simulink model "RB_KAIROS_impControl_repulsive"  (R2020b)
settings: Solver=ode4  StartTime=0.0  StopTime=t_end  FixedStep=Ts  RelTol=1e-3
values from neighbouring files (symbols this model uses):
  am = 0.3    [RB_KAIROS_ImpControl_OpSpace_quat_2020b_safety_main.m]
  am_r = 0.3    [RB_KAIROS_ImpControl_OpSpace_quat_2020b_safety_main.m]
  Kc = diag(50*ones(6,1))    [RB_KAIROS_ImpControl_OpSpace_quat_2020b_safety_main.m]
  Kp = 2*[400;400;400;400;0;0;0]    [RB_KAIROS_ImpControl_OpSpace_quat_2020b_safety_main.m]
  Kv = [1000;1000;1000;[300;300;300;300;300;300;300]]    [RB_KAIROS_ImpControl_OpSpace_quat_2020b_safety_main.m]
  model_sample_time = 0.001    [RB_KAIROS_ImpControl_OpSpace_quat_2020b_safety_main.m]
  q_dot_0 = zeros(10,1)    [RB_KAIROS_ImpControl_OpSpace_quat_2020b_safety_main.m]
  T_i = K    [RB_KAIROS_ImpControl_OpSpace_quat_2020b_safety_main.m]
  tau_ext = [0 0 0 0 0 0 0 0 0 0 0]    [RB_KAIROS_ImpControl_OpSpace_quat_2020b_safety_main.m]
  v_SMU = 10    [RB_KAIROS_ImpControl_OpSpace_quat_2020b_safety_main.m]
  vm = 0.5    [RB_KAIROS_ImpControl_OpSpace_quat_2020b_safety_main.m]
  vm_r = 0.5    [RB_KAIROS_ImpControl_OpSpace_quat_2020b_safety_main.m]
undefined symbols (not defined in the file or in its folder): DiscIntNeverNeededParam, magnitude, q_0, T_f
libraries: simulink x4, utils x4, transformations_lib x3
(part 14 of 17)

== matlab function RB_KAIROS_impControl_repulsive/CONTROLLER /Kinematics and Dynamics/Kinematics - error representation/MATLAB Function1 ==
  data: J input; t output
function t = fcn(J)

t = 0;
%you can use normc(J) to see if one column gets near 0 and by this you get
%directions that are singular
D = sqrt(det(J*J'));
if(D < 10e-2)
    t = 1;
    disp(J)
end

== matlab function RB_KAIROS_impControl_repulsive/Trajectory Generator/Subsystem1/MATLAB Function ==
  data: u input; y output
function y = fcn(u)

y = rotm2eul(u, 'XYZ')';

== matlab function RB_KAIROS_impControl_repulsive/CONTROLLER /Kinematics and Dynamics/Kinematics - error representation/MATLAB Function2 ==
  data: R_D_W_aug input; vt output; x_dot_d input; x_ddot_d input; vt_dot output; x_err input; x_dot_err input
function [vt, vt_dot] = compute_vt(R_D_W_aug, x_dot_d, x_ddot_d, x_err, x_dot_err)
% This function is used to compute the vectors vt and vt_dot defined in Ott book in order
% to convert the equation of motion to an equivalent representation using
% error on the task variables

% INPUTS:
% - R_W_D_aug is an extension of the ROTATION MATRIX from world frame to 
%   desired frame: [R_W_D 0; 0 R_W_D], it is a 6x6 matrix
% - omega_d, p_dot_d, p_err, eps_err, omega_err are all quantities defined in
%   the world frame (or space frame) W.
S_omega_d = calc_skewsymm(x_dot_d(4:6));
S_alfa_d = calc_skewsymm(x_ddot_d(4:6));

a = [x_dot_d(1:3) + S_omega_d*(x_err(1:3));
                x_dot_d(4:6)];

vt = R_D_W_aug*a;

vt_dot = R_D_W_aug*(-augment_matrix(S_omega_d)*a + [x_ddot_d(1:3) + S_alfa_d*x_err(1:3) + S_omega_d*x_dot_err(1:3);
                                                                  x_ddot_d(4:6)]);

end 


function S = calc_skewsymm(v)

S = [0 -v(3) v(2);
    v(3) 0 -v(1);
    -v(2) v(1) 0];
end

function M_aug = augment_matrix(M)

M_aug = [M, zeros(3,3);
             zeros(3,3), M];
end

== matlab function RB_KAIROS_impControl_repulsive/CONTROLLER /Kinematics and Dynamics/Kinematics - error representation/MATLAB Function3 ==
  data: R_W_D_aug input; J_x output; J_b input
function J_x   =compute_J_x(R_W_D_aug, J_b)
% This function is used to compute the matrix J_x defined in Ott book in order
% to convert the equation of motion to an equivalent representation using
% error on the task variables

% INPUTS:
% - R_W_D_aug is an extension of the ROTATION MATRIX from world frame to 
%   desired frame: [R_W_D 0; 0 R_W_D], it is a 6x6 matrix
% - J_b is the body Jacobian of the robot 

J_x = R_W_D_aug*J_b;

== matlab function RB_KAIROS_impControl_repulsive/CONTROLLER /Kinematics and Dynamics/Kinematics - error representation/Whole-Body Jacobian ==
  data: qv input; J output size=[6,10]; qa input
function J = get_J(qv,qa)
%GET_J
%    J = GET_J(qv,qa)

%    This function was generated by the Symbolic Math Toolbox version 8.6.
%    14-Feb-2023 10:02:51

phi = qv(3);

q1 = qa(1);
q2 = qa(2);
q3 = qa(3);
q4 = qa(4);
q5 = qa(5);
q6 = qa(6);
t2 = cos(phi);
t3 = cos(q1);
t4 = cos(q2);
t5 = cos(q3);
t6 = cos(q4);
t7 = cos(q5);
t8 = cos(q6);
t9 = sin(phi);
t10 = sin(q1);
t11 = sin(q2);
t12 = sin(q3);
t13 = sin(q4);
t14 = sin(q5);
t15 = sin(q6);
t16 = t3.*t5;
t17 = t4.*t6;
t18 = t3.*t12;
t19 = t5.*t10;
t20 = t4.*t13;
t21 = t10.*t12;
t22 = -t9;
t23 = t10.*t11.*t13;
t24 = t11.*t12.*t14;
t28 = t3.*t6.*t11;
t29 = t5.*t6.*t11;
t31 = t3.*t11.*t13;
t32 = t6.*t10.*t11;
t33 = t5.*t11.*t13;
t34 = t7.*t11.*t12;
t41 = t4.*(7.9e+1./2.5e+2);
t44 = t5.*t11.*(3.3e+1./4.0e+2);
t47 = t3.*t11.*(7.9e+1./2.5e+2);
t50 = t10.*t11.*(7.9e+1./2.5e+2);
t124 = t2.*1.224646799147353e-16;
t125 = t9.*1.224646799147353e-16;
t138 = t3.*t11.*3.869883885305636e-17;
t139 = t10.*t11.*3.869883885305636e-17;
t25 = t4.*t16;
t26 = t4.*t18;
t27 = t4.*t19;
t30 = t4.*t21;
t36 = -t29;
t38 = -t31;
t39 = -t32;
t40 = -t34;
t42 = t17.*(4.8e+1./1.25e+2);
t43 = t18.*(3.3e+1./4.0e+2);
t45 = t20.*(3.3e+1./4.0e+2);
t46 = t21.*(3.3e+1./4.0e+2);
t48 = -t44;
t52 = t23.*(3.3e+1./4.0e+2);
t55 = t17+t33;
t57 = t28.*(4.8e+1./1.25e+2);
t59 = t29.*(3.3e+1./4.0e+2);
t60 = t32.*(4.8e+1./1.25e+2);
t61 = t33.*(4.8e+1./1.25e+2);
t62 = t31.*(3.3e+1./4.0e+2);
t127 = t2+t125;
t130 = t22+t124;
t132 = t28.*4.702643708725836e-17;
t133 = t32.*4.702643708725836e-17;
t136 = t18.*1.010333609296566e-17;
t137 = t21.*1.010333609296566e-17;
t141 = -t138;
t144 = t31.*1.010333609296566e-17;
t145 = t23.*1.010333609296566e-17;
t35 = -t25;
t37 = -t30;
t49 = -t45;
t51 = -t46;
t53 = t18+t27;
t54 = t19+t26;
t56 = t25.*(3.3e+1./4.0e+2);
t58 = t27.*(3.3e+1./4.0e+2);
t63 = -t52;
t65 = -t57;
t66 = -t62;
t69 = t20+t36;
t72 = t8.*t55;
t85 = t15.*t55.*(1.1e+1./1.25e+2);
t135 = -t132;
t142 = t25.*1.010333609296566e-17;
t143 = t27.*1.010333609296566e-17;
t147 = -t145;
t64 = -t56;
t67 = t16+t37;
t68 = t21+t35;
t70 = t6.*t53;
t71 = t7.*t54;
t73 = t13.*t53;
t74 = t14.*t54;
t78 = t7.*t69;
t79 = -t72;
t82 = t14.*t69;
t91 = t72.*(1.07e+2./1.0e+3);
t146 = -t142;
t75 = t6.*t68;
t76 = t7.*t67;
t77 = -t71;
t80 = t13.*t68;
t81 = t14.*t67;
t84 = t70.*(3.3e+1./4.0e+2);
t86 = t73.*(4.8e+1./1.25e+2);
t89 = t23+t70;
t94 = -t91;
t96 = t39+t73;
t97 = t24+t78;
t101 = t40+t82;
t104 = -t8.*(t32-t73);
t110 = t15.*(t32-t73).*(-1.1e+1./1.25e+2);
t112 = t15.*(t32-t73).*(1.1e+1./1.25e+2);
t114 = t8.*(t32-t73).*(-1.07e+2./1.0e+3);
t149 = t73.*4.702643708725836e-17;
t152 = t70.*1.010333609296566e-17;
t159 = t15.*(t32-t73).*(-1.077689183249671e-17);
t162 = t15.*(t32-t73).*1.077689183249671e-17;
t164 = t8.*(t32-t73).*(-1.310372075087668e-17);
t83 = -t76;
t87 = -t84;
t88 = -t86;
t90 = t75.*(3.3e+1./4.0e+2);
t92 = t80.*(4.8e+1./1.25e+2);
t98 = t28+t80;
t99 = t7.*t89;
t100 = t14.*t89;
t102 = t38+t75;
t105 = t15.*t97;
t106 = -t7.*(t31-t75);
t107 = -t14.*(t31-t75);
t109 = t8.*t97.*(1.1e+1./1.25e+2);
t150 = -t149;
t151 = t80.*4.702643708725836e-17;
t154 = -t152;
t155 = t75.*1.010333609296566e-17;
t93 = -t90;
t95 = -t92;
t103 = t8.*t98;
t108 = t15.*t98.*(1.1e+1./1.25e+2);
t115 = t105.*(1.07e+2./1.0e+3);
t117 = t81+t99;
t118 = t74+t106;
t119 = t83+t100;
t120 = t79+t105;
t122 = t77+t107;
t153 = -t151;
t156 = -t155;
t158 = t15.*t98.*1.077689183249671e-17;
t111 = -t108;
t113 = t103.*(1.07e+2./1.0e+3);
t121 = t15.*t117;
t123 = t15.*t118;
t126 = t8.*t117.*(1.1e+1./1.25e+2);
t128 = t8.*t118.*(1.1e+1./1.25e+2);
t148 = t94+t115;
t161 = -t158;
t163 = t103.*1.310372075087668e-17;
t167 = t8.*t117.*1.077689183249671e-17;
t168 = t8.*t118.*1.077689183249671e-17;
t116 = -t113;
t129 = t121.*(1.07e+2./1.0e+3);
t131 = -t128;
t134 = t123.*(1.07e+2./1.0e+3);
t157 = t104+t121;
t160 = t103+t123;
t169 = t121.*1.310372075087668e-17;
t170 = t123.*1.310372075087668e-17;
t171 = t85+t109+t148;
t140 = -t134;
t165 = t114+t129;
t166 = t113+t134;
t172 = -t157.*(t91-t115);
t174 = -t160.*(t91-t115);
t177 = t98.*t171;
t178 = -t171.*(t32-t73);
t180 = t42+t49+t59+t61+t171;
t181 = -t171.*(t76-t100);
t182 = -t171.*(t71+t14.*(t31-t75));
t183 = t171.*(t76-t100);
t199 = -t11.*t12.*(t52-t60+t84+t86+t110-t126-t129+t8.*(t32-t73).*(1.07e+2./1.0e+3));
t200 = t11.*t12.*(t52-t60+t84+t86+t110-t126-t129+t8.*(t32-t73).*(1.07e+2./1.0e+3));
t173 = -t165.*(t72-t105);
t175 = -t166.*(t72-t105);
t176 = t165.*(t72-t105);
t179 = t166.*(t72-t105);
t184 = t48+t180;
t185 = t54.*t180;
t186 = t67.*t180;
t189 = t112+t126+t165;
t191 = t111+t128+t166;
t202 = -t11.*t12.*(t57+t66+t90+t92+t108+t116+t131+t140);
t203 = t11.*t12.*(t57+t66+t90+t92+t108+t116+t131+t140);
t210 = -t4.*(t51+t56+t57+t66+t90+t92+t108+t116+t131+t140);
t211 = t47+t51+t56+t57+t66+t90+t92+t108+t116+t131+t140;
t187 = t3.*t11.*t184;
t188 = t10.*t11.*t184;
t192 = t41+t184;
t193 = t55.*t189;
t194 = t55.*t191;
t195 = -t189.*(t34-t82);
t196 = -t191.*(t34-t82);
t197 = t191.*(t34-t82);
t198 = t60+t63+t87+t88+t189;
t201 = t62+t65+t93+t95+t191;
t206 = t172+t176;
t208 = t174+t179;
t216 = t186+t200;
t217 = t185+t203;
t220 = t133+t136+t139+t143+t147+t150+t154+t162+t164+t167+t169+t211+1.1e+1./4.0e+1;
t190 = -t188;
t204 = t43+t58+t198;
t207 = t46+t64+t201;
t212 = t178+t193;
t213 = t177+t194;
t214 = t183+t195;
t215 = t182+t197;
t219 = t187+t210;
t205 = t4.*t204;
t209 = t50+t204;
t218 = t190+t205;
t221 = t135+t137+t141+t144+t146+t153+t156+t161+t163+t168+t170+t209+3.1e+1./2.0e+2;
J = reshape([1.0,0.0,0.0,0.0,0.0,0.0,0.0,1.0,0.0,0.0,0.0,0.0,t2.*t221+t9.*t220,-t2.*t220+t9.*t221,0.0,0.0,0.0,1.0,t127.*t209-t130.*t211,-t127.*t211-t130.*t209,0.0,0.0,0.0,1.0,-t3.*t127.*t192-t10.*t130.*t192,t3.*t130.*t192-t10.*t127.*t192,-t3.*t211-t10.*t209,-t3.*t130+t10.*t127,-t3.*t127-t10.*t130,0.0,t130.*t219-t127.*(t188-t205),t127.*t219+t130.*(t188-t205),-t10.*t11.*(t51+t56+t57+t66+t90+t92+t108+t116+t131+t140)+t3.*t11.*t204,-t3.*t11.*t127-t10.*t11.*t130,t3.*t11.*t130-t10.*t11.*t127,t4,t127.*t216+t130.*t217,t127.*t217-t130.*t216,t67.*(t57+t66+t90+t92+t108+t116+t131+t140)-t54.*(t52-t60+t84+t86+t110-t126-t129+t8.*(t32-t73).*(1.07e+2./1.0e+3)),-t54.*t127+t67.*t130,t54.*t130+t67.*t127,-t11.*t12,t127.*(t193-t171.*(t32-t73))+t130.*t213,-t130.*(t193-t171.*(t32-t73))+t127.*t213,t98.*t189+t191.*(t32-t73),-t98.*t127-t130.*(t32-t73),t98.*t130-t127.*(t32-t73),t55,t127.*t214+t130.*(t196+t171.*(t71+t14.*(t31-t75))),-t130.*t214+t127.*(t196+t171.*(t71+t14.*(t31-t75))),t189.*(t71+t14.*(t31-t75))-t191.*(t76-t100),-t127.*(t71+t14.*(t31-t75))+t130.*(t76-t100),t130.*(t71+t14.*(t31-t75))+t127.*(t76-t100),t101,-t127.*t206-t130.*t208,-t127.*t208+t130.*t206,t157.*t166-t160.*t165,t127.*t160-t130.*t157,-t127.*t157-t130.*t160,t120],[6,10]);

== matlab function RB_KAIROS_impControl_repulsive/CONTROLLER /MATLAB Function ==
  data: qa_des input; qa_des_new output; qv input
function qa_des_new = fcn(qa_des,qv)

qa_des_new = qa_des;
% qa_des_new(1) = qa_des_new(1)+qv(3);

== matlab function RB_KAIROS_impControl_repulsive/CONTROLLER /Primary task - Controller/MATLAB Function ==
  data: Kc input; Dc output; Lambda input
function Dc = compute_damping(Kc,Lambda)
%  COMPUTE_DAMPING Computes damping matrix to enforce desired second order
%  system behaviour.
%
%   Dc = COMPUTE_DAMPING(Kc,Lambda) computes the damping depending on 
%        stiffness matrix Kc (which has to be constant for stability) and
%        inertia matrix Lambda (which is time varying since no inertia 
%        shaping is applied).
%   
%   Reference: Cartesian Impedance Control of Redundant and Flexible-Joint
%              Robots, C. Ott 2005, page 36-37.
%   See also EIG

% % DAMPING MATRIX (varying) simplified
zeta = 1*ones(6,1);

A = real(sqrtm(Lambda));
Kc_1 = real(sqrtm(Kc));
D0 = diag(zeta);
Dc = A*D0*Kc_1 + Kc_1*D0*A;

% DAMPING MATRIX (varying)
%Generalized eigenvalue decomposition for the pair (Kc,Lambda)
% [eigvecs,eigvals] = eig(Kc, Lambda);
% eigvals = real(eigvals);
% eigvecs = real(eigvecs);
% %sorting eigs by magnitude
% %[eigvals,sidx] = sort(diag(eigvals),'descend');
% 
% %Finding matrices that satisfy K = Q'K0Q and Lambda = Q'*Q
% K0 = eigvals;
% %V = eigvecs(:,sidx);
% Q_T = Lambda*eigvecs;
% Q = Q_T';
% 
% %Damping matrix computation
% zeta = 1*ones(6,1); %Imposing an overdamped behaviour
% D0 = diag(zeta).*K0;
% Dc = 2*Q_T*D0*Q;

%OLD implementation where stiffness and damping were retrieven from
%configuration parameters
%function [Kc,Dc] = compute_stiffness_damping(J, J_T, J_i, J_d, Lambda)

% Kq_veh = [750*ones(2,1); 750]; 
% Dq_veh = [800;800;800];
% Kq_arm = [350;250;100;170;50;20;10];
% Dq_arm = [60;200;120;150;20;30;5];
% 
% Kq = diag([Kq_veh;Kq_arm]);
% Dq = diag([Dq_veh;Dq_arm]);
% 
% Dc = J_i'*Dq*J_i;
% Kc = J_i'*(Kq-J_T*Dc*J_d)*J_i;

% Kc = diag([150;180;105;1.5;15;52.5]);
% Dc = diag([180;200;80;10;10;6]);

== matlab function RB_KAIROS_impControl_repulsive/CONTROLLER /Secondary task - Controller/MATLAB Function ==
  data: qa_des input; qa input; tau_n output; qa_dot input; qv_dot input; M input; J_x_T input; J_x_i input; Kp input; Kv input
function tau_n = compute_null_space_torque(qa_des, qa, qa_dot, qv_dot, M, J_x_T, J_x_i, Kp, Kv)


%% Version 1: Try to keep the robot joints in their mid position
% q_max = [2.3093; 1.5133; 2.4937; -0.4461; 2.4800; 4.2094; 2.6895];
% q_min = [-2.3093; -1.5133; -2.4937; -2.7478; -2.4800; 0.8521; -2.6895];
% tau_0 = -M*[Kv(1:3).*qv_dot;2*Kp.*(qa-(q_max+q_min)./2)+Kv(4:10).*qa_dot];
% Good but the mid config. of every joint is not super good for any motion

%% Version 2: Mantain a certain configuration 
%Compute generalized joint torque based on the gradient of the potential
%that is used to mantain a certain configuration of the arm.

    tau_0 = -M*[Kv(1:3).*qv_dot;
         Kp.*(qa-qa_des)+Kv(4:10).*qa_dot]; 
    

%% Projection of the torque in the null space
tau_n = (eye(size(M,2))-J_x_T*J_x_i')*tau_0;

== matlab function RB_KAIROS_impControl_repulsive/EE to task space quaternion quantities/Augment matrix ==
  data: R_W_D input; R_D_W_aug output
function R_D_W_aug = augment_matrix(R_W_D)

R_D_W_aug = [R_W_D', zeros(3,3);
             zeros(3,3), R_W_D'];

== matlab function RB_KAIROS_impControl_repulsive/EE to task space quaternion quantities/Get Pose in quaternions ==
  data: T_W_EE input; p_EE output; qt_EE output
function [p_EE, qt_EE] = tform2pose_quat(T_W_EE)
% Retrieves the pose of the end effector using quaternion representation
% for the orientation 

p_EE = T_W_EE(1:3,4);
qt_EE = tform2quat(T_W_EE)';

== matlab function RB_KAIROS_impControl_repulsive/Trajectory Generator/move2pose/Cartesian_ipol2/rotation/Embedded MATLAB Function1 ==
  data: t input; qd output; s0 input; v0 input; sf input; vm input; am input; dqd output; ddqd output; ipol_finished output; T_scale input; interpoly input
function [qd,dqd,ddqd, ipol_finished] = calc_qd(t,s0,v0,sf,vm,am,T_scale,interpoly)
% This function calculates a one dimensional movement with a trapezodial 
% signal for velocity over time. Additionally it is able to adapt to shifts
% in the maximum allowed velocity.
%
% Inputs:
% t         current runtime
% s0        start value for motion in position
% v0        start value for motion in velocity
% sf        final value for motion in position
% vm        maximum allowed velocity
% am        maximum allowed acceleration
% T_scale   Scaling factor for duration of adaption
% interpoly Which interpolation to use
%
% Outputs:
% qd        disered position at current time
% dqd       disered velocity at current time
% ddqd      disered acceleration at current time
% ipol_finished 
%           motion is finished

%% Initialize persistent variables for adaption motion
persistent vm1 adpt ti qi qf T t_shift
if isempty(vm1)
    vm1 = vm;       %remembers the max velocity from last run
end
if isempty(adpt)
    adpt = false;   %stores if an adaption motion is activated
end
if isempty(ti)
    ti = 0;         %Initial time step for adaption motion
end
if isempty(qi)
    qi = zeros(3,1);%Initial values (pos,vel,acc) for adaption motion
end
if isempty(qf)
    qf = zeros(3,1);%Final values (pos,vel,acc) for adaption motion
end
if isempty(T)
    T = 0;          %Duration of adaption motion; tf = ti+T
end
if isempty(t_shift)
    t_shift = 0;    %Time distance with which the current reference motion is shifted
end

% needed to delay tanhlog with one timestep
tanhlog_delay = 0;

%% This If runs only for one timestep!!!
% If current max velocity is unequal to old one 
% Not directly at the beginning
% Dont start new while a adaption is still running, to prevent reset of
%   initial values
if abs(vm-vm1)>1e-3 && t>0.001 && adpt==false                       
    adpt = true;          % Activate adaption
    ti = t;               % Set initial timestep to current step
    tanhlog_delay = 1;    % Activate the delay for tanhlog

    %%% inital set of position, velo, acceleration for adaption motion 
    % is the same as the old mogen would do (t_shift is not updated at
    % this time!)
    [qi, ~] = interpolator(ti+t_shift, compute_traj_parameters(s0, v0, sf, vm1, am));

    %%% computes the time shift for shifting the new motion to the end
    % point of the old motion. So at which time the new motion has
    % the same qd? Then calculate the time distance to the inital
    % time of the change in velocities
    % t_shift < 0 if new motion is faster (vm>vm1)
    % t_shift > 0 if new motion is slower (vm<vm1)
    % interpolator_1 is the inverse function of interpolator!
    t_shift = interpolator_1(qi(1), compute_traj_parameters(s0, v0, sf, vm, am)) - ti ;

    %%% Additional shift for adaption motion = Duration of adaption motion
    T_standard = abs(vm1-vm)/am;
    switch interpoly
        case 0
            T = 0;
            adpt = false;       %no adatption  
        case 1
            T = T_standard*2.2;    %tanhlog
        case 2
            T = (pi*abs(vm1-vm))/(2*am);  %Cosine version
        case 3
            T = T_standard;        %poly3
        case 4
            T = 1.5*(abs(vm1-vm)/am); %poly4
        case 5
            T = T_standard*1.5;        %poly5 
        case 7
            T = T_standard*1.75;        %poly7 
        otherwise
            T = T_standard;        %rest
    end

    % Scale Duration if needed
    T = T*T_scale;

    %%% The additional shift for adaption motion is dependent on the
    % difference in the velocities. See report for details.
    t_shift  = t_shift+(T/2)*((vm1/vm)-1);

    %%% Calculate final values for adaption motion. Which are reached
    % at inital time plus duration of adaption and new time shift
    [qf, ~] = interpolator(ti+t_shift+T, compute_traj_parameters(s0, v0, sf, vm, am));

end

%% Here the actual motion is calculated
% Interpolates the values of pos,vel,acc (qv) with parameters and current time t    
[qdv, ipol_finished] = interpolator(t+t_shift, compute_traj_parameters(s0, v0, sf, vm, am));  

%% If adaption motion needed
if adpt == true 

    %%% calculate the adaption moition, which takes time from ti to
    % ti+T. t is the current runtime, _i initial values, _f final
    % values, _m maximum values

    switch interpoly
        case 0
            adpt=false;                             %no adatption  
        case 1
            if tanhlog_delay == 1
                qdv = qi;  
                tanhlog_delay = 0;
            else
                qdv = tanhlog(t,ti,T,qi,qf,vm,am);      %tanhlog
            end
        case 2
            qdv = cosine(t,ti,T,qi,qf,vm,am);       %Cosine version
        case 3
            qdv = poly3(t,ti,T,qi,qf,vm,am);        %poly3
        case 4
            qdv = poly4(t,ti,T,qi,qf,vm,am);        %poly4
        case 5
            qdv = poly5(t,ti,T,qi,qf,vm,am);        %poly5 
        case 6
            qdv = poly6(t,ti,T,qi,qf,vm,am);        %poly6 
        case 7
            qdv = poly7(t,ti,T,qi,qf,vm,am);        %poly7 
        case 8
            qdv = poly4_mean(t,ti,T,qi,qf,vm,am);   %poly4_mean 
        case 9
            qdv = poly5_2mean(t,ti,T,qi,qf,vm,am);  %poly5_2mean 
        case 10
            qdv = tanhmean(t,ti,T,qi,qf,vm,am);     %tanhmean 
        otherwise
            error('Unknown adaption motion');       %rest
    end

    % If time is equal than the finish time => adaption motion is complete
    % But it is aborted one timestep earlier, since the finish timestep
    % is already computed correctly by the standard interpolator.
    if t >= (ti+T-0.001)
        adpt = false;     % If adaption finished => reset
    end
end

%% Set output
if sf == s0          % No motion needed if start = end 
    qd = s0;         % => set initial values
    dqd = v0;
    ddqd = 0;  
else     
    qd = qdv(1);     % set output
    dqd = qdv(2);
    ddqd = qdv(3);        
end

vm1 = vm;  %remember current max velocity

end

function [qv] = poly3(t,ti,T,qvi,qvf,dqm,ddqm)
%POLY3 computes a polynomial trajectory of degree 3 between initial (_i) 
%values and final (_f) values of position q, velocity dq and accelerataion
%ddq. Taken from Melchiorri presentation page 19

qi = qvi(1);      %split input vectors in pos,vel,acc
dqi = qvi(2);
ddqi = qvi(3);
qf = qvf(1);
dqf = qvf(2);
ddqf = qvf(3);
      
% current duration of motion dt
dt = t-ti;                      

% compute coefficients
a0 = qi;
a1 = dqi;
a2 = (-3*(qi-qf)-(2*dqi+dqf)*T)/(T^2);
a3 = (2*(qi-qf)+(dqi+dqf)*T)/(T^3);

% compute pos,vel,acc desired (_d)
qd = a0+a1*dt+a2*dt^2+a3*dt^3;
dqd = a1+2*a2*dt+3*a3*dt^2;
ddqd = 2*a2+6*a3*dt;

qv = [qd;dqd;ddqd]; %Send values back

end

function [qv] = poly4(t,ti,T,qvi,qvf,dqm,ddqm)
%POLY4 computes a polynomial trajectory of degree 4 between initial (_i) 
%values and final (_f) values of position q, velocity dq and accelerataion
%ddq. inspired by old function in here

qi = qvi(1);      %split input vectors in pos,vel,acc
dqi = qvi(2);
ddqi = qvi(3);
qf = qvf(1);
dqf = qvf(2);
ddqf = qvf(3);
      
% current duration of motion dt
dt = t-ti;                      

% a2 = 0;
% a3 = -4/9*ddqm^2/(dqi-dqm);
% a4 = -4/27*ddqm^3/(dqi-dqm)^2;
a2 = 0;
a3 = -4/9*ddqm^2/abs(dqi-dqf);
a4 = 4/27*ddqm^3/abs(dqi-dqf)^2;

a0 = qi;
a1 = dqi;
% a2 = 0.5*ddqi;
% a3 = (4*(qf-qi)-(dqf+3*dqi)*T-ddqi*(T^2))/(T^3);
% a4 = (3*(qi-qf)+(dqf+2*dqi)*T+0.5*ddqi*(T^2))/(T^4);

% compute pos,vel,acc desired (_d)
qd = (a4*dt^4+a3*dt^3+a2*dt^2+a1*dt+a0);
dqd = 4*a4*dt^3+3*a3*dt^2+2*a2*dt+a1;
ddqd = 12*a4*dt^2+6*a3*dt+2*a2;

qv = [qd;dqd;ddqd]; %Send values back

end

function [qv] = poly4_mean(t,ti,T,qvi,qvf,dqm,ddqm)
%POLY4 computes a polynomial trajectory of degree 4 between initial (_i) 
%values and final (_f) values of position q, velocity dq and accelerataion
%ddq with mean velocity at T/2. self made

qi = qvi(1);      %split input vectors in pos,vel,acc
dqi = qvi(2);
ddqi = qvi(3);
qf = qvf(1);
dqf = qvf(2);
ddqf = qvf(3);
      
% current duration of motion dt
dt = t-ti;                     

b = [qi dqi qf dqf 0.5*(dqi+dqf)]';

M_inv = [...
       1,     0,      0,          0,           0;
       0,     1,      0,          0,           0;
   6/T^2,  -2/T, -6/T^2,    5/(4*T),    27/(4*T);
 -16/T^3, 1/T^2, 16/T^3, -7/(2*T^2), -27/(2*T^2);
   9/T^4,     0, -9/T^4,  9/(4*T^3),  27/(4*T^3)];

a = M_inv * b;

% compute pos,vel,acc desired (_d)

qd = a(1)+a(2)*dt+a(3)*dt^2+a(4)*dt^3+a(5)*dt^4;
dqd = a(2)+2*a(3)*dt+3*a(4)*dt^2+4*a(5)*dt^3;
ddqd = 2*a(3)+6*a(4)*dt+12*a(5)*dt^2;

qv = [qd;dqd;ddqd]; %Send values back

end

function [qv] = poly5(t,ti,T,qvi,qvf,dqm,ddqm)
%POLY5 computes a polynomial trajectory of degree 5 between initial (_i) 
%values and final (_f) values of position q, velocity dq and accelerataion
%ddq. Taken from Melchiorri presentation page 25

qi = qvi(1);      %split input vectors in pos,vel,acc
dqi = qvi(2);
ddqi = qvi(3);
qf = qvf(1);
dqf = qvf(2);
ddqf = qvf(3);
      
% current duration of motion dt
dt = t-ti;                      

% compute coefficients
a0 = qi;
a1 = dqi;
a2 = 0.5*ddqi;
a3 = (20*(qf-qi)-(8*dqf+12*dqi)*T-(3*ddqf-ddqi)*T^2)/(2*T^3);
a4 = (30*(qi-qf)+(14*dqf+16*dqi)*T+(3*ddqf-2*ddqi)*T^2)/(2*T^4);
a5 = (12*(qf-qi)-6*(dqf+dqi)*T-(ddqf-ddqi)*T^2)/(2*T^5);

% compute pos,vel,acc desired (_d)
qd = a0+a1*dt+a2*dt^2+a3*dt^3+a4*dt^4+a5*dt^5;
dqd = a1+2*a2*dt+3*a3*dt^2+4*a4*dt^3+5*a5*dt^4;
ddqd = 2*a2+6*a3*dt+12*a4*dt^2+20*a5*dt^3;

qv = [qd;dqd;ddqd]; %Send values back

end

function [qv] = poly5_2mean(t,ti,T,qvi,qvf,dqm,ddqm)
%POLY5 computes a polynomial trajectory of degree 5 between initial (_i) 
%values and final (_f) values of position q, velocity dq and accelerataion
%ddq with 2*mean steps at T/3 and 2T/3. self made

qi = qvi(1);      %split input vectors in pos,vel,acc
dqi = qvi(2);
ddqi = qvi(3);
qf = qvf(1);
dqf = qvf(2);
ddqf = qvf(3);
      
% current duration of motion dt
dt = t-ti;                      

% compute coefficients
b = [qi dqi qf dqf 0.5*(dqi+dqf)+(1/6)*(dqi-dqf) 0.5*(dqi+dqf)+(1/6)*(dqi-dqf)]';

M_inv = [...
        1,          0,        0,           0,            0,           0;
        0,          1,        0,           0,            0,           0;
  -30/T^2,  -13/(2*T),   30/T^2,   -13/(4*T),    -27/(4*T),   -27/(2*T);
  110/T^3, 67/(4*T^2), -110/T^3,  49/(4*T^2),  135/(4*T^2), 189/(4*T^2);
 -135/T^4,    -18/T^3,  135/T^4, -63/(4*T^3), -189/(4*T^3),     -54/T^3;
   54/T^5, 27/(4*T^4),  -54/T^5,  27/(4*T^4),   81/(4*T^4),  81/(4*T^4)];

a = M_inv * b;

% compute pos,vel,acc desired (_d)

qd = a(1)+a(2)*dt+a(3)*dt^2+a(4)*dt^3+a(5)*dt^4+a(6)*dt^5;
dqd = a(2)+2*a(3)*dt+3*a(4)*dt^2+4*a(5)*dt^3+5*a(6)*dt^4;
ddqd = 2*a(3)+6*a(4)*dt+12*a(5)*dt^2+20*a(6)*dt^3;

qv = [qd;dqd;ddqd]; %Send values back

end

function [qv] = poly6(t,ti,T,qvi,qvf,dqm,ddqm)
%POLY6 computes a polynomial trajectory of degree 6 between initial (_i) 
%values and final (_f) values of position q, velocity dq and accelerataion
%ddq with mean velocity at T/3. self made

qi = qvi(1);      %split input vectors in pos,vel,acc
dqi = qvi(2);
ddqi = qvi(3);
qf = qvf(1);
dqf = qvf(2);
ddqf = qvf(3);

% current duration of motion dt
dt = t-ti;                      

% compute coefficients
b = [qi dqi 0.5*ddqi qf dqf ddqf 0.5*(dqi+dqf)]';

M_inv = [...
       1,      0,      0,       0,           0,          0,            0;
       0,      1,      0,       0,           0,          0,            0;
       0,      0,      1,       0,           0,          0,            0;
  20/T^3, -6/T^2,   -4/T, -20/T^3,  23/(4*T^2),   -1/(2*T),   81/(4*T^2);
 -75/T^4,  8/T^3,  6/T^2,  75/T^4, -89/(4*T^3),      2/T^2, -243/(4*T^3);
  84/T^5, -3/T^4, -4/T^3, -84/T^5, 105/(4*T^4), -5/(2*T^3),  243/(4*T^4);
 -30/T^6,      0,  1/T^4,  30/T^6, -39/(4*T^5),      1/T^4,  -81/(4*T^5)];

a = M_inv * b;

% compute pos,vel,acc desired (_d)

qd = a(1)+a(2)*dt+a(3)*dt^2+a(4)*dt^3+a(5)*dt^4+a(6)*dt^5+a(7)*dt^6;
dqd = a(2)+2*a(3)*dt+3*a(4)*dt^2+4*a(5)*dt^3+5*a(6)*dt^4+6*a(7)*dt^5;
ddqd = 2*a(3)+6*a(4)*dt+12*a(5)*dt^2+20*a(6)*dt^3+30*a(7)*dt^4;

qv = [qd;dqd;ddqd]; %Send values back

end

function [qv] = poly7(t,ti,T,qvi,qvf,dqm,ddqm)
%POLY7 computes a polynomial trajectory of degree 7 between initial (_i) 
%values and final (_f) values of position q, velocity dq, accelerataion
%ddq and jerk dddq. self made

qi = qvi(1);      %split input vectors in pos,vel,acc
dqi = qvi(2);
ddqi = qvi(3);
dddqi = 0;
qf = qvf(1);
dqf = qvf(2);
ddqf = qvf(3);
dddqf = 0;

% current duration of motion dt
dt = t-ti;                      

% compute coefficients
 
a = [...
                                                                                                                                                                            conj(qi)
                                                                                                                                                                           conj(dqi)
                                                                                                                                                                        conj(ddqi)/2
                                                                                                                                                                       conj(dddqi)/6
           (5*conj(ddqf))/(2*T^2) - (2*conj(dddqi))/(3*T) - conj(dddqf)/(6*T) - (5*conj(ddqi))/T^2 - (15*conj(dqf))/T^3 - (20*conj(dqi))/T^3 + (35*conj(qf))/T^4 - (35*conj(qi))/T^4
                  conj(dddqf)/(2*T^2) + conj(dddqi)/T^2 - (7*conj(ddqf))/T^3 + (10*conj(ddqi))/T^3 + (39*conj(dqf))/T^4 + (45*conj(dqi))/T^4 - (84*conj(qf))/T^5 + (84*conj(qi))/T^5
 (13*conj(ddqf))/(2*T^4) - (2*conj(dddqi))/(3*T^3) - conj(dddqf)/(2*T^3) - (15*conj(ddqi))/(2*T^4) - (34*conj(dqf))/T^5 - (36*conj(dqi))/T^5 + (70*conj(qf))/T^6 - (70*conj(qi))/T^6
               conj(dddqf)/(6*T^4) + conj(dddqi)/(6*T^4) - (2*conj(ddqf))/T^5 + (2*conj(ddqi))/T^5 + (10*conj(dqf))/T^6 + (10*conj(dqi))/T^6 - (20*conj(qf))/T^7 + (20*conj(qi))/T^7];
 


% compute pos,vel,acc desired (_d)

qd = a(1)+a(2)*dt+a(3)*dt^2+a(4)*dt^3+a(5)*dt^4+a(6)*dt^5+a(7)*dt^6+a(8)*dt^7;
dqd = a(2)+2*a(3)*dt+3*a(4)*dt^2+4*a(5)*dt^3+5*a(6)*dt^4+6*a(7)*dt^5+7*a(8)*dt^6;
ddqd = 2*a(3)+6*a(4)*dt+12*a(5)*dt^2+20*a(6)*dt^3+30*a(7)*dt^4+42*a(8)*dt^5;

qv = [qd;dqd;ddqd]; %Send values back

end

function [qv] = cosine(t,ti,T,qvi,qvf,dqm,ddqm)
%COSINE computes a cosine trajectory between initial (_i) 
%values and final (_f) values of position q, velocity dq and accelerataion
%ddq with respect to the maximum values (_m). t is the current runtime

qi = qvi(1);      %split input vectors in pos,vel,acc
dqi = qvi(2);
ddqi = qvi(3);
qf = qvf(1);
dqf = qvf(2);
ddqf = qvf(3);
      
% often needed values

%T = (pi*abs(dqf-dqi))/(2*ddqm); % total duration of motion T (with am)
%T = abs((2*(qf-qi))/(dqi-dqf));
dt = t-ti;                      % current duration of motion dt

%cm = (T/(2*pi))*(dqm-(1/T)*(qf-qi));
c = qi-0.5*(dqi+dqf)*ti;
%cn = qf-0.5*(dqi+dqf)*(ti+T);
%c = cn + 0.5*(1+cos((pi/T)*dt))*(ca-cn);


% if t<(ti+(T/2))
%     c = qi - 0.5*(dqi+dqf)*ti;
% else
%     c = qf - 0.5*(((dqi+dqf)/2)+dqf)*tf;
% end

%c = (qi+qf)/2 - 0.5*(dqi+dqf)*(ti+(T/2)) - 0.5*(dqi-dqf)*(T/pi);
% compute pos,vel,acc desired (_d)
%qd = qi + (1/T)*(qf-qi)*dt + cm*sin(((2*pi)/T)*dt);
qd = 0.5*(dqi+dqf)*t + 0.5*(T/pi)*(dqi-dqf)*sin((pi/T)*dt) + c;
dqd = 0.5*(dqi+dqf) + 0.5*(dqi-dqf)*cos((pi/T)*dt);
ddqd = -0.5*(pi/T)*(dqi-dqf)*sin((pi/T)*dt);

qv = [qd;dqd;ddqd]; %Send values back

end

function [qv] = tanhmean(t,ti,T,qvi,qvf,dqm,ddqm)
%TANHMEAN computes a tanh trajectory between initial (_i) 
%values and final (_f) values of position q, velocity dq and accelerataion
%ddq with respect to the maximum values (_m). t is the current runtime
%selfmade

qi = qvi(1);      %split input vectors in pos,vel,acc
dqi = qvi(2);
ddqi = qvi(3);
qf = qvf(1);
dqf = qvf(2);
ddqf = qvf(3);
      
% current duration of motion dt
dt = t-ti;                      
t_norm = dt/T;
theta = 4;

qd = 0.5*(1/theta)*(dqf-dqi)*log(cosh(theta*(t_norm-0.5))) ...
     + 0.5*(dqi+dqf)*t_norm ...
     + qf - 0.5*(1/theta)*(dqf-dqi)*log(cosh(0.5*theta));
     %+ qi - 0.5*(1/theta)*(dqf-dqi)*log(cosh(-0.5*theta));
dqd = 0.5*(dqi+dqf) + 0.5*(dqf-dqi)*tanh(theta*(t_norm-0.5));
ddqd = 0.5*theta*(dqf-dqi)*sech(t_norm-0.5)^2;

qv = [qd;dqd;ddqd]; %Send values back

end

function [qv] = tanhlog(t,ti,T,qvi,qvf,dqm,ddqm)
%TANHLOG computes a tanh-log trajectory between initial (_i) 
%values and final (_f) values of position q, velocity dq and accelerataion
%ddq with respect to the maximum values (_m). t is the current runtime
%taken from Internet

qi = qvi(1);      %split input vectors in pos,vel,acc
dqi = qvi(2);
ddqi = qvi(3);
qf = qvf(1);
dqf = qvf(2);
ddqf = qvf(3);
      
% current duration of motion dt
dt = t-ti;  

a = dqi;
b = qi;      
c = dqf;
d = qf-dqf*T;
k = d-b;

x = (a*dt+b-c*dt-d+k)/(2*k);
w = (tanh(((log(1-x))^2-(log(x))^2)/3)+1)/2;
p = tanh((log(2-x)-log(x))*(1-(1/sqrt(2))*(log(2-x)+log(x))))+2*x-1;
q = tanh((log(x+1)-log(1-x))*(1-(1/sqrt(2))*(log(1-x)+log(x+1))));
s = p*(1-w)+q*w;

qd = k*s+c*dt+d-k;

dqd = dqf + (qi - qf + T*dqf)*((tanh(log((dqf*dt - dqi*dt)/(2*qi - 2*qf + 2*T*dqf))^2/3 - log(1 - (dqf*dt - dqi*dt)/(2*qi - 2*qf + 2*T*dqf))^2/3)/2 + 1/2)*((((2^(1/2)*(log(2 - (dqf*dt - dqi*dt)/(2*qi - 2*qf + 2*T*dqf)) + log((dqf*dt - dqi*dt)/(2*qi - 2*qf + 2*T*dqf))))/2 - 1)*((dqf - dqi)/(dqf*dt - dqi*dt) - (dqf - dqi)/(((dqf*dt - dqi*dt)/(2*qi - 2*qf + 2*T*dqf) - 2)*(2*qi - 2*qf + 2*T*dqf))) - (2^(1/2)*(log(2 - (dqf*dt - dqi*dt)/(2*qi - 2*qf + 2*T*dqf)) - log((dqf*dt - dqi*dt)/(2*qi - 2*qf + 2*T*dqf)))*((dqf - dqi)/(dqf*dt - dqi*dt) + (dqf - dqi)/(((dqf*dt - dqi*dt)/(2*qi - 2*qf + 2*T*dqf) - 2)*(2*qi - 2*qf + 2*T*dqf))))/2)*(tanh((log(2 - (dqf*dt - dqi*dt)/(2*qi - 2*qf + 2*T*dqf)) - log((dqf*dt - dqi*dt)/(2*qi - 2*qf + 2*T*dqf)))*((2^(1/2)*(log(2 - (dqf*dt - dqi*dt)/(2*qi - 2*qf + 2*T*dqf)) + log((dqf*dt - dqi*dt)/(2*qi - 2*qf + 2*T*dqf))))/2 - 1))^2 - 1) - (2*(dqf - dqi))/(2*qi - 2*qf + 2*T*dqf)) - (tanh(((2^(1/2)*(log((dqf*dt - dqi*dt)/(2*qi - 2*qf + 2*T*dqf) + 1) + log(1 - (dqf*dt - dqi*dt)/(2*qi - 2*qf + 2*T*dqf))))/2 - 1)*(log((dqf*dt - dqi*dt)/(2*qi - 2*qf + 2*T*dqf) + 1) - log(1 - (dqf*dt - dqi*dt)/(2*qi - 2*qf + 2*T*dqf))))^2 - 1)*(tanh(log((dqf*dt - dqi*dt)/(2*qi - 2*qf + 2*T*dqf))^2/3 - log(1 - (dqf*dt - dqi*dt)/(2*qi - 2*qf + 2*T*dqf))^2/3)/2 - 1/2)*(((2^(1/2)*(log((dqf*dt - dqi*dt)/(2*qi - 2*qf + 2*T*dqf) + 1) + log(1 - (dqf*dt - dqi*dt)/(2*qi - 2*qf + 2*T*dqf))))/2 - 1)*((dqf - dqi)/(((dqf*dt - dqi*dt)/(2*qi - 2*qf + 2*T*dqf) - 1)*(2*qi - 2*qf + 2*T*dqf)) - (dqf - dqi)/(((dqf*dt - dqi*dt)/(2*qi - 2*qf + 2*T*dqf) + 1)*(2*qi - 2*qf + 2*T*dqf))) - (2^(1/2)*(log((dqf*dt - dqi*dt)/(2*qi - 2*qf + 2*T*dqf) + 1) - log(1 - (dqf*dt - dqi*dt)/(2*qi - 2*qf + 2*T*dqf)))*((dqf - dqi)/(((dqf*dt - dqi*dt)/(2*qi - 2*qf + 2*T*dqf) - 1)*(2*qi - 2*qf + 2*T*dqf)) + (dqf - dqi)/(((dqf*dt - dqi*dt)/(2*qi - 2*qf + 2*T*dqf) + 1)*(2*qi - 2*qf + 2*T*dqf))))/2) + (tanh(((2^(1/2)*(log((dqf*dt - dqi*dt)/(2*qi - 2*qf + 2*T*dqf) + 1) + log(1 - (dqf*dt - dqi*dt)/(2*qi - 2*qf + 2*T*dqf))))/2 - 1)*(log((dqf*dt - dqi*dt)/(2*qi - 2*qf + 2*T*dqf) + 1) - log(1 - (dqf*dt - dqi*dt)/(2*qi - 2*qf + 2*T*dqf))))*((2*log((dqf*dt - dqi*dt)/(2*qi - 2*qf + 2*T*dqf))*(dqf - dqi))/(3*(dqf*dt - dqi*dt)) - (2*log(1 - (dqf*dt - dqi*dt)/(2*qi - 2*qf + 2*T*dqf))*(dqf - dqi))/(3*((dqf*dt - dqi*dt)/(2*qi - 2*qf + 2*T*dqf) - 1)*(2*qi - 2*qf + 2*T*dqf)))*(tanh(log((dqf*dt - dqi*dt)/(2*qi - 2*qf + 2*T*dqf))^2/3 - log(1 - (dqf*dt - dqi*dt)/(2*qi - 2*qf + 2*T*dqf))^2/3)^2 - 1))/2 - (((2*log((dqf*dt - dqi*dt)/(2*qi - 2*qf + 2*T*dqf))*(dqf - dqi))/(3*(dqf*dt - dqi*dt)) - (2*log(1 - (dqf*dt - dqi*dt)/(2*qi - 2*qf + 2*T*dqf))*(dqf - dqi))/(3*((dqf*dt - dqi*dt)/(2*qi - 2*qf + 2*T*dqf) - 1)*(2*qi - 2*qf + 2*T*dqf)))*(tanh(log((dqf*dt - dqi*dt)/(2*qi - 2*qf + 2*T*dqf))^2/3 - log(1 - (dqf*dt - dqi*dt)/(2*qi - 2*qf + 2*T*dqf))^2/3)^2 - 1)*(tanh((log(2 - (dqf*dt - dqi*dt)/(2*qi - 2*qf + 2*T*dqf)) - log((dqf*dt - dqi*dt)/(2*qi - 2*qf + 2*T*dqf)))*((2^(1/2)*(log(2 - (dqf*dt - dqi*dt)/(2*qi - 2*qf + 2*T*dqf)) + log((dqf*dt - dqi*dt)/(2*qi - 2*qf + 2*T*dqf))))/2 - 1)) - (2*(dqf*dt - dqi*dt))/(2*qi - 2*qf + 2*T*dqf) + 1))/2);

ddqd = -(qi - qf + T*dqf)*(((tanh(log((dqf*dt - dqi*dt)/(2*qi - 2*qf + 2*T*dqf))^2/3 - log(1 - (dqf*dt - dqi*dt)/(2*qi - 2*qf + 2*T*dqf))^2/3)^2 - 1)*(tanh((log(2 - (dqf*dt - dqi*dt)/(2*qi - 2*qf + 2*T*dqf)) - log((dqf*dt - dqi*dt)/(2*qi - 2*qf + 2*T*dqf)))*((2^(1/2)*(log(2 - (dqf*dt - dqi*dt)/(2*qi - 2*qf + 2*T*dqf)) + log((dqf*dt - dqi*dt)/(2*qi - 2*qf + 2*T*dqf))))/2 - 1)) - (2*(dqf*dt - dqi*dt))/(2*qi - 2*qf + 2*T*dqf) + 1)*((2*(dqf - dqi)^2)/(3*(dqf*dt - dqi*dt)^2) - (2*(dqf - dqi)^2)/(3*((dqf*dt - dqi*dt)/(2*qi - 2*qf + 2*T*dqf) - 1)^2*(2*qi - 2*qf + 2*T*dqf)^2) - (2*log((dqf*dt - dqi*dt)/(2*qi - 2*qf + 2*T*dqf))*(dqf - dqi)^2)/(3*(dqf*dt - dqi*dt)^2) + (2*log(1 - (dqf*dt - dqi*dt)/(2*qi - 2*qf + 2*T*dqf))*(dqf - dqi)^2)/(3*((dqf*dt - dqi*dt)/(2*qi - 2*qf + 2*T*dqf) - 1)^2*(2*qi - 2*qf + 2*T*dqf)^2)))/2 - (tanh(((2^(1/2)*(log((dqf*dt - dqi*dt)/(2*qi - 2*qf + 2*T*dqf) + 1) + log(1 - (dqf*dt - dqi*dt)/(2*qi - 2*qf + 2*T*dqf))))/2 - 1)*(log((dqf*dt - dqi*dt)/(2*qi - 2*qf + 2*T*dqf) + 1) - log(1 - (dqf*dt - dqi*dt)/(2*qi - 2*qf + 2*T*dqf))))*(tanh(log((dqf*dt - dqi*dt)/(2*qi - 2*qf + 2*T*dqf))^2/3 - log(1 - (dqf*dt - dqi*dt)/(2*qi - 2*qf + 2*T*dqf))^2/3)^2 - 1)*((2*(dqf - dqi)^2)/(3*(dqf*dt - dqi*dt)^2) - (2*(dqf - dqi)^2)/(3*((dqf*dt - dqi*dt)/(2*qi - 2*qf + 2*T*dqf) - 1)^2*(2*qi - 2*qf + 2*T*dqf)^2) - (2*log((dqf*dt - dqi*dt)/(2*qi - 2*qf + 2*T*dqf))*(dqf - dqi)^2)/(3*(dqf*dt - dqi*dt)^2) + (2*log(1 - (dqf*dt - dqi*dt)/(2*qi - 2*qf + 2*T*dqf))*(dqf - dqi)^2)/(3*((dqf*dt - dqi*dt)/(2*qi - 2*qf + 2*T*dqf) - 1)^2*(2*qi - 2*qf + 2*T*dqf)^2)))/2 - (tanh(log((dqf*dt - dqi*dt)/(2*qi - 2*qf + 2*T*dqf))^2/3 - log(1 - (dqf*dt - dqi*dt)/(2*qi - 2*qf + 2*T*dqf))^2/3)/2 + 1/2)*((tanh((log(2 - (dqf*dt - dqi*dt)/(2*qi - 2*qf + 2*T*dqf)) - log((dqf*dt - dqi ...
    *dt)/(2*qi - 2*qf + 2*T*dqf)))*((2^(1/2)*(log(2 - (dqf*dt - dqi*dt)/(2*qi - 2*qf + 2*T*dqf)) + log((dqf*dt - dqi*dt)/(2*qi - 2*qf + 2*T*dqf))))/2 - 1))^2 - 1)*((2^(1/2)*(log(2 - (dqf*dt - dqi*dt)/(2*qi - 2*qf + 2*T*dqf)) - log((dqf*dt - dqi*dt)/(2*qi - 2*qf + 2*T*dqf)))*((dqf - dqi)^2/(dqf*dt - dqi*dt)^2 + (dqf - dqi)^2/(((dqf*dt - dqi*dt)/(2*qi - 2*qf + 2*T*dqf) - 2)^2*(2*qi - 2*qf + 2*T*dqf)^2)))/2 - ((dqf - dqi)^2/(dqf*dt - dqi*dt)^2 - (dqf - dqi)^2/(((dqf*dt - dqi*dt)/(2*qi - 2*qf + 2*T*dqf) - 2)^2*(2*qi - 2*qf + 2*T*dqf)^2))*((2^(1/2)*(log(2 - (dqf*dt - dqi*dt)/(2*qi - 2*qf + 2*T*dqf)) + log((dqf*dt - dqi*dt)/(2*qi - 2*qf + 2*T*dqf))))/2 - 1) + 2^(1/2)*((dqf - dqi)/(dqf*dt - dqi*dt) + (dqf - dqi)/(((dqf*dt - dqi*dt)/(2*qi - 2*qf + 2*T*dqf) - 2)*(2*qi - 2*qf + 2*T*dqf)))*((dqf - dqi)/(dqf*dt - dqi*dt) - (dqf - dqi)/(((dqf*dt - dqi*dt)/(2*qi - 2*qf + 2*T*dqf) - 2)*(2*qi - 2*qf + 2*T*dqf)))) + 2*tanh((log(2 - (dqf*dt - dqi*dt)/(2*qi - 2*qf + 2*T*dqf)) - log((dqf*dt - dqi*dt)/(2*qi - 2*qf + 2*T*dqf)))*((2^(1/2)*(log(2 - (dqf*dt - dqi*dt)/(2*qi - 2*qf + 2*T*dqf)) + log((dqf*dt - dqi*dt)/(2*qi - 2*qf + 2*T*dqf))))/2 - 1))*(((2^(1/2)*(log(2 - (dqf*dt - dqi*dt)/(2*qi - 2*qf + 2*T*dqf)) + log((dqf*dt - dqi*dt)/(2*qi - 2*qf + 2*T*dqf))))/2 - 1)*((dqf - dqi)/(dqf*dt - dqi*dt) - (dqf - dqi)/(((dqf*dt - dqi*dt)/(2*qi - 2*qf + 2*T*dqf) - 2)*(2*qi - 2*qf + 2*T*dqf))) - (2^(1/2)*(log(2 - (dqf*dt - dqi*dt)/(2*qi - 2*qf + 2*T*dqf)) - log((dqf*dt - dqi*dt)/(2*qi - 2*qf + 2*T*dqf)))*((dqf - dqi)/(dqf*dt - dqi*dt) + (dqf - dqi)/(((dqf*dt - dqi*dt)/(2*qi - 2*qf + 2*T*dqf) - 2)*(2*qi - 2*qf + 2*T*dqf))))/2)^2*(tanh((log(2 - (dqf*dt - dqi*dt)/(2*qi - 2*qf + 2*T*dqf)) - log((dqf*dt - dqi*dt)/(2*qi - 2*qf + 2*T*dqf)))*((2^(1/2)*(log(2 - (dqf*dt - dqi*dt)/(2*qi - 2*qf + 2*T*dqf)) + log((dqf*dt - dqi*dt)/(2*qi - 2*qf + 2*T*dqf))))/2 - 1))^2 - 1)) + ((2*log((dqf*dt - dqi*dt)/(2*qi - 2*qf + 2*T*dqf))*(dqf - dqi))/(3*(dqf*dt - dqi*dt)) - (2*log(1 - (dqf*dt - dqi*dt)/(2*qi - 2*qf + 2*T*dqf))*(dqf - dqi))/(3*((dqf*dt - dqi*dt)/(2*qi - 2*qf + 2*T*dqf) - 1)*(2*qi - 2*qf + 2*T*dqf)))*(tanh(log((dqf*dt - dqi*dt)/(2*qi - 2*qf + 2*T*dqf))^2/3 - log(1 - (dqf*dt - dqi*dt)/(2*qi - 2*qf + 2*T*dqf))^2/3)^2 - 1)*((((2^(1/2)*(log(2 - (dqf*dt - dqi*dt)/(2*qi - 2*qf + 2*T*dqf)) + log((dqf*dt - dqi*dt)/(2*qi - 2*qf + 2*T*dqf))))/2 - 1)*((dqf - dqi)/(dqf*dt - dqi*dt) - (dqf - dqi)/(((dqf*dt - dqi*dt)/(2*qi - 2*qf + 2*T*dqf) - 2)*(2*qi - 2*qf + 2*T*dqf))) - (2^(1/2)*(log(2 - (dqf*dt - dqi*dt)/(2*qi - 2*qf + 2*T*dqf)) - log((dqf*dt - dqi*dt)/(2*qi - 2*qf + 2*T*dqf)))*((dqf - dqi)/(dqf*dt - dqi*dt) + (dqf - dqi)/(((dqf*dt - dqi*dt)/(2*qi - 2*qf + 2*T*dqf) - 2)*(2*qi - 2*qf + 2*T*dqf))))/2)*(tanh((log(2 - (dqf*dt - dqi*dt)/(2*qi - 2*qf + 2*T*dqf)) - log((dqf*dt - dqi*dt)/(2*qi - 2*qf + 2*T*dqf)))*((2^(1/2)*(log(2 - (dqf*dt - dqi*dt)/(2*qi - 2*qf + 2*T*dqf)) + log((dqf*dt - dqi*dt)/(2*qi - 2*qf + 2*T*dqf))))/2 - 1))^2 - 1) - (2*(dqf - dqi))/(2*qi - 2*qf + 2*T*dqf)) + (tanh(((2^(1/2)*(log((dqf*dt - dqi*dt)/(2*qi - 2*qf + 2*T*dqf) + 1) + log(1 - (dqf*dt - dqi*dt)/(2*qi - 2*qf + 2*T*dqf))))/2 - 1)*(log((dqf*dt - dqi*dt)/(2*qi - 2*qf + 2*T*dqf) + 1) - log(1 - (dqf*dt - dqi*dt)/(2*qi - 2*qf + 2*T*dqf))))^2 - 1)*(tanh(log((dqf*dt - dqi*dt)/(2*qi - 2*qf + 2*T*dqf))^2/3 - log(1 - (dqf*dt - dqi*dt)/(2*qi - 2*qf + 2*T*dqf))^2/3)/2 - 1/2)*(2^(1/2)*((dqf - dqi)/(((dqf*dt - dqi*dt)/(2*qi - 2*qf + 2*T*dqf) - 1)*(2*qi - 2*qf + 2*T*dqf)) + (dqf - dqi)/(((dqf*dt - dqi*dt)/(2*qi - 2*qf + 2*T*dqf) + 1)*(2*qi - 2*qf + 2*T*dqf)))*((dqf - dqi)/(((dqf*dt - dqi*dt)/(2*qi - 2*qf + 2*T*dqf) - 1) ...
    *(2*qi - 2*qf + 2*T*dqf)) - (dqf - dqi)/(((dqf*dt - dqi*dt)/(2*qi - 2*qf + 2*T*dqf) + 1)*(2*qi - 2*qf + 2*T*dqf))) - ((2^(1/2)*(log((dqf*dt - dqi*dt)/(2*qi - 2*qf + 2*T*dqf) + 1) + log(1 - (dqf*dt - dqi*dt)/(2*qi - 2*qf + 2*T*dqf))))/2 - 1)*((dqf - dqi)^2/(((dqf*dt - dqi*dt)/(2*qi - 2*qf + 2*T*dqf) - 1)^2*(2*qi - 2*qf + 2*T*dqf)^2) - (dqf - dqi)^2/(((dqf*dt - dqi*dt)/(2*qi - 2*qf + 2*T*dqf) + 1)^2*(2*qi - 2*qf + 2*T*dqf)^2)) + (2^(1/2)*(log((dqf*dt - dqi*dt)/(2*qi - 2*qf + 2*T*dqf) + 1) - log(1 - (dqf*dt - dqi*dt)/(2*qi - 2*qf + 2*T*dqf)))*((dqf - dqi)^2/(((dqf*dt - dqi*dt)/(2*qi - 2*qf + 2*T*dqf) - 1)^2*(2*qi - 2*qf + 2*T*dqf)^2) + (dqf - dqi)^2/(((dqf*dt - dqi*dt)/(2*qi - 2*qf + 2*T*dqf) + 1)^2*(2*qi - 2*qf + 2*T*dqf)^2)))/2) + tanh(((2^(1/2)*(log((dqf*dt - dqi*dt)/(2*qi - 2*qf + 2*T*dqf) + 1) + log(1 - (dqf*dt - dqi*dt)/(2*qi - 2*qf + 2*T*dqf))))/2 - 1)*(log((dqf*dt - dqi*dt)/(2*qi - 2*qf + 2*T*dqf) + 1) - log(1 - (dqf*dt - dqi*dt)/(2*qi - 2*qf + 2*T*dqf))))*tanh(log((dqf*dt - dqi*dt)/(2*qi - 2*qf + 2*T*dqf))^2/3 - log(1 - (dqf*dt - dqi*dt)/(2*qi - 2*qf + 2*T*dqf))^2/3)*((2*log((dqf*dt - dqi*dt)/(2*qi - 2*qf + 2*T*dqf))*(dqf - dqi))/(3*(dqf*dt - dqi*dt)) - (2*log(1 - (dqf*dt - dqi*dt)/(2*qi - 2*qf + 2*T*dqf))*(dqf - dqi))/(3*((dqf*dt - dqi*dt)/(2*qi - 2*qf + 2*T*dqf) - 1)*(2*qi - 2*qf + 2*T*dqf)))^2*(tanh(log((dqf*dt - dqi*dt)/(2*qi - 2*qf + 2*T*dqf))^2/3 - log(1 - (dqf*dt - dqi*dt)/(2*qi - 2*qf + 2*T*dqf))^2/3)^2 - 1) - (tanh(((2^(1/2)*(log((dqf*dt - dqi*dt)/(2*qi - 2*qf + 2*T*dqf) + 1) + log(1 - (dqf*dt - dqi*dt)/(2*qi - 2*qf + 2*T*dqf))))/2 - 1)*(log((dqf*dt - dqi*dt)/(2*qi - 2*qf + 2*T*dqf) + 1) - log(1 - (dqf*dt - dqi*dt)/(2*qi - 2*qf + 2*T*dqf))))^2 - 1)*((2*log((dqf*dt - dqi*dt)/(2*qi - 2*qf + 2*T*dqf))*(dqf - dqi))/(3*(dqf*dt - dqi*dt)) - (2*log(1 - (dqf*dt - dqi*dt)/(2*qi - 2*qf + 2*T*dqf))*(dqf - dqi))/(3*((dqf*dt - dqi*dt)/(2*qi - 2*qf + 2*T*dqf) - 1)*(2*qi - 2*qf + 2*T*dqf)))*(tanh(log((dqf*dt - dqi*dt)/(2*qi - 2*qf + 2*T*dqf))^2/3 - log(1 - (dqf*dt - dqi*dt)/(2*qi - 2*qf + 2*T*dqf))^2/3)^2 - 1)*(((2^(1/2)*(log((dqf*dt - dqi*dt)/(2*qi - 2*qf + 2*T*dqf) + 1) + log(1 - (dqf*dt - dqi*dt)/(2*qi - 2*qf + 2*T*dqf))))/2 - 1)*((dqf - dqi)/(((dqf*dt - dqi*dt)/(2*qi - 2*qf + 2*T*dqf) - 1)*(2*qi - 2*qf + 2*T*dqf)) - (dqf - dqi)/(((dqf*dt - dqi*dt)/(2*qi - 2*qf + 2*T*dqf) + 1)*(2*qi - 2*qf + 2*T*dqf))) - (2^(1/2)*(log((dqf*dt - dqi*dt)/(2*qi - 2*qf + 2*T*dqf) + 1) - log(1 - (dqf*dt - dqi*dt)/(2*qi - 2*qf + 2*T*dqf)))*((dqf - dqi)/(((dqf*dt - dqi*dt)/(2*qi - 2*qf + 2*T*dqf) - 1)*(2*qi - 2*qf + 2*T*dqf)) + (dqf - dqi)/(((dqf*dt - dqi*dt)/(2*qi - 2*qf + 2*T*dqf) + 1)*(2*qi - 2*qf + 2*T*dqf))))/2) - tanh(log((dqf*dt - dqi*dt)/(2*qi - 2*qf + 2*T*dqf))^2/3 - log(1 - (dqf*dt - dqi*dt)/(2*qi - 2*qf + 2*T*dqf))^2/3)*((2*log((dqf*dt - dqi*dt)/(2*qi - 2*qf + 2*T*dqf))*(dqf - dqi))/(3*(dqf*dt - ...
    dqi*dt)) - (2*log(1 - (dqf*dt - dqi*dt)/(2*qi - 2*qf + 2*T*dqf))*(dqf - dqi))/(3*((dqf*dt - dqi*dt)/(2*qi - 2*qf + 2*T*dqf) - 1)*(2*qi - 2*qf + 2*T*dqf)))^2*(tanh(log((dqf*dt - dqi*dt)/(2*qi - 2*qf + 2*T*dqf))^2/3 - log(1 - (dqf*dt - dqi*dt)/(2*qi - 2*qf + 2*T*dqf))^2/3)^2 - 1)*(tanh((log(2 - (dqf*dt - dqi*dt)/(2*qi - 2*qf + 2*T*dqf)) - log((dqf*dt - dqi*dt)/(2*qi - 2*qf + 2*T*dqf)))*((2^(1/2)*(log(2 - (dqf*dt - dqi*dt)/(2*qi - 2*qf + 2*T*dqf)) + log((dqf*dt - dqi*dt)/(2*qi - 2*qf + 2*T*dqf))))/2 - 1)) - (2*(dqf*dt - dqi*dt))/(2*qi - 2*qf + 2*T*dqf) + 1) + 2*tanh(((2^(1/2)*(log((dqf*dt - dqi*dt)/(2*qi - 2*qf + 2*T*dqf) + 1) + log(1 - (dqf*dt - dqi*dt)/(2*qi - 2*qf + 2*T*dqf))))/2 - 1)*(log((dqf*dt - dqi*dt)/(2*qi - 2*qf + 2*T*dqf) + 1) - log(1 - (dqf*dt - dqi*dt)/(2*qi - 2*qf + 2*T*dqf))))*(tanh(((2^(1/2)*(log((dqf*dt - dqi*dt)/(2*qi - 2*qf + 2*T*dqf) + 1) + log(1 - (dqf*dt - dqi*dt)/(2*qi - 2*qf + 2*T*dqf))))/2 - 1)*(log((dqf*dt - dqi*dt)/(2*qi - 2*qf + 2*T*dqf) + 1) - log(1 - (dqf*dt - dqi*dt)/(2*qi - 2*qf + 2*T*dqf))))^2 - 1)*(tanh(log((dqf*dt - dqi*dt)/(2*qi - 2*qf + 2*T*dqf))^2/3 - log(1 - (dqf*dt - dqi*dt)/(2*qi - 2*qf + 2*T*dqf))^2/3)/2 - 1/2)*(((2^(1/2)*(log((dqf*dt - dqi*dt)/(2*qi - 2*qf + 2*T*dqf) + 1) + log(1 - (dqf*dt - dqi*dt)/(2*qi - 2*qf + 2*T*dqf))))/2 - 1)*((dqf - dqi)/(((dqf*dt - dqi*dt)/(2*qi - 2*qf + 2*T*dqf) - 1)*(2*qi - 2*qf + 2*T*dqf)) - (dqf - dqi)/(((dqf*dt - dqi*dt)/(2*qi - 2*qf + 2*T*dqf) + 1)*(2*qi - 2*qf + 2*T*dqf))) - (2^(1/2)*(log((dqf*dt - dqi*dt)/(2*qi - 2*qf + 2*T*dqf) + 1) - log(1 - (dqf*dt - dqi*dt)/(2*qi - 2*qf + 2*T*dqf)))*((dqf - dqi)/(((dqf*dt - dqi*dt)/(2*qi - 2*qf + 2*T*dqf) - 1)*(2*qi - 2*qf + 2*T*dqf)) + (dqf - dqi)/(((dqf*dt - dqi*dt)/(2*qi - 2*qf + 2*T*dqf) + 1)*(2*qi - 2*qf + 2*T*dqf))))/2)^2);

qv = [qd;dqd;ddqd]; %Send values back

end

function ris=compute_traj_parameters(s0, v0, sf, vm, am)
    ris=zeros(15,1);
    radix=zeros(2,1);
    T1 = 0;
    dT = 0;
    T2 = 0;
    a1 = 0;
    b1 = 0;
    c1 = 0;
    d1 = 0;
    e1 = 0;
    a2 = 0;
    b2 = 0;
    c2 = 0;
    d2 = 0;
    e2 = 0;
    k = 0;

    if (vm~=0) %check...
        vm=vm*sign(sf-s0);
        k=am*sign(sf-s0);
        T1 = -3/2*(v0-vm)/k;
        a1 = -4/27*k^3/(v0-vm)^2;
        b1 = -4/9*k^2/(v0-vm);
        e1 = s0;
        d1 = v0;
        c1 = 0;
        c2 = 0;
        T2 = 3/2*vm/k;
        dT = 1/4*(-3*vm^2+4*sf*k-4*a1*T1^4*k-4*b1*T1^3*k-4*c1*T1^2*k-4*d1*T1*k-4*e1*k)/vm/k;
        a2 = 4/27*k^3/vm^2;
        d2 = vm;
        e2 = 1/4*(-3*vm^2+4*sf*k)/k;
        b2 = -4/9*k^2/vm;
        if (dT<0)
            c2 = 0;
            c1 = 0;
            a=2;
            b=12*v0;
            c=9*v0^2-12*sf*k+12*s0*k;
            radix(1)=(-b + sqrt(b^2-4*a*c))/(2*a);
            radix(2)=(-b - sqrt(b^2-4*a*c))/(2*a);
            %decide the correct root
            T1_a = 1/2*radix(1)/k;
            T2_a = 1/2*(radix(1)+3*v0)/k;
            T1_b = 1/2*radix(2)/k;
            T2_b = 1/2*(radix(2)+3*v0)/k;
                if (and(T1_a>=0, T2_a>=0))
                    r=radix(1);
                    T1=T1_a;
                    T2=T2_a;
                    dT=0;
                    two_phases=1;
                elseif (and(T1_b>=0, T2_b>=0))
                    r=radix(2);
                    T1=T1_b;
                    T2=T2_b;
                    dT=0;
                    two_phases=1;
                else
                    r=0;
                    two_phases=0;
                end
                if (two_phases==0)
                    T1=0;
                    T2=2*(sf-s0)/v0;
                    dT=0;
                    b2=-1/4*v0^3/(sf-s0)^2;
                    c2=0;
                    a2=1/16*v0^4/(sf-s0)^3;
                    d2=v0;
                    e2=s0;
                else
                    b1 = -8/9*k^2/(4*v0*r+3*v0^2-4*sf*k+4*s0*k)*r;
                    a1 = 8/9*k^3/(4*v0*r+3*v0^2-4*sf*k+4*s0*k);
                    b2 = -8/9*k^2/(4*sf*k+3*v0^2-4*s0*k)*(r+3*v0);
                    e2 = -1/8*(3*v0^2-4*s0*k-4*sf*k)/k;
                    e1 = s0;
                    d1 = v0;
                    d2 = 2/9/(4*sf*k+3*v0^2-4*s0*k)*(r+3*v0)^3;
                    a2 = 8/9*k^3/(4*sf*k+3*v0^2-4*s0*k);
                end
        end
    end
    ris=[T1;dT;T2; a1; b1; c1; d1; e1; a2; b2; c2; d2; e2; vm; k];
end

%time, and the output of the previous function
function [ris, finished]=interpolator(t, parameters)

ris=zeros(3,1);
T1=parameters(1);
dT=parameters(2);
T2=parameters(3);
a1=parameters(4);
b1=parameters(5);
c1=parameters(6);
d1=parameters(7);
e1=parameters(8);
a2=parameters(9);
b2=parameters(10);
c2=parameters(11);
d2=parameters(12);
e2=parameters(13);
vm=parameters(14);
k=parameters(15);

finished = 0;
if (vm~=0) %check...
        if (t<=T1)
            ris=[a1*t^4+b1*t^3+c1*t^2+d1*t+e1; 4*a1*t^3+3*b1*t^2+2*c1*t+d1; 12*a1*t^2+6*b1*t+2*c1];
        elseif (t<=T1+dT)
            t=t-T1;
            ris=[a1*T1^4+b1*T1^3+c1*T1^2+d1*T1+e1+vm*t; vm; 0];
        elseif (t<=T1+dT+T2)
            t=t-T1-dT;
            ris=[a2*t^4+b2*t^3+c2*t^2+d2*t+e2; 4*a2*t^3+3*b2*t^2+2*c2*t+d2; 12*a2*t^2+6*b2*t+2*c2];
        else
            t=T2;
            ris=[a2*t^4+b2*t^3+c2*t^2+d2*t+e2;0;0];
            finished=1;
        end
else
    ris=[0;0;0];
end

end

function t=interpolator_1(q, parameters)

T1=parameters(1);
dT=parameters(2);
T2=parameters(3);
a1=parameters(4);
b1=parameters(5);
c1=parameters(6);
d1=parameters(7);
e1=parameters(8);
a2=parameters(9);
b2=parameters(10);
c2=parameters(11);
d2=parameters(12);
e2=parameters(13);
vm=parameters(14);
k=parameters(15);

t=0;
Q1 = a1*T1^4+b1*T1^3+c1*T1^2+d1*T1+e1;%q point at end of startup
Q2 = a2*T2^4+b2*T2^3+c2*T2^2+d2*T2+e2;%final q
Q3 = Q2-Q1;%q point at end of linear part (using symmetry)

if q<Q1
    %startup
%     %tarray = 0:0.001:T1; %not working, because T1 should be constant?!
%     tarray = linspace(0,T1);
%     qarray=zeros(size(tarray));
%     parfor i=1:size(tarray,2)
%         [qv,~]=interpolator(tarray(i), parameters);
%         qarray(i)=qv(1);
%     end
%     t = interp1(qarray, tarray, q);
    t=0;
    error('trans: interpolator_1 startup: not programmed jet, sry');
    % problem with calculating additional shift
elseif q>=Q1 || q<=Q3
    %linear part
    t = T1+((q-Q1)/vm);
elseif q>Q3
    %slowdown
    t=0;
    error('trans: interpolator_1 slowdown: not programmed jet, sry');
end

end

== matlab function RB_KAIROS_impControl_repulsive/EE to task space quaternion quantities/MATLAB Function ==
  data: qt input; qt_unit output
function qt_unit = qt_norm(qt)

qt_unit = qt./norm(qt);
